simulink model "examen_simulacion_11_01_2024"  (R2024a)
settings: Solver=FixedStepAuto  StartTime=0.0  StopTime=10  FixedStep=0.01  RelTol=1e-3
values from neighbouring files (symbols this model uses):
  a_adelanto = y + Pd1_real    [examen_11_01_2024.m]
  a_adelanto2 = y2 + Pd1_real    [examen_11_01_2024.m]
  b_adelanto = abs(real(polos_LA(3)))    [examen_11_01_2024.m]
  b_adelanto2 = abs(real(polos_LA(2)))    [examen_11_01_2024.m]
  G_den = den    [examen_11_01_2024.m]
  G_num = num    [examen_11_01_2024.m]
  ganancias = 15:2:25    [examen_11_01_2024.m]
undefined symbols (not defined in the file or in its folder): K_rlocfind, K_rlocfind2
libraries: simulink x1
settings Model: Creator=david  LastModifiedBy=david

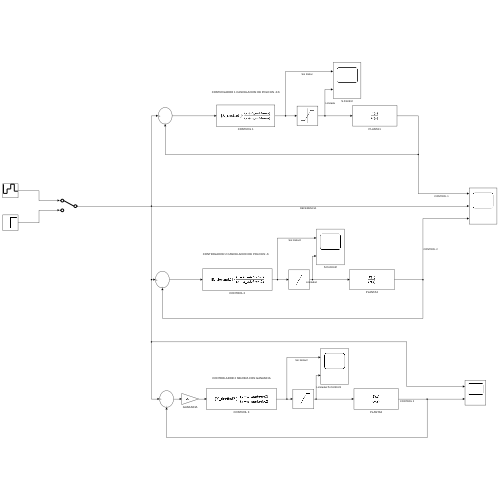
[thumbnail: Simulink's stored preview of the top-level diagram]
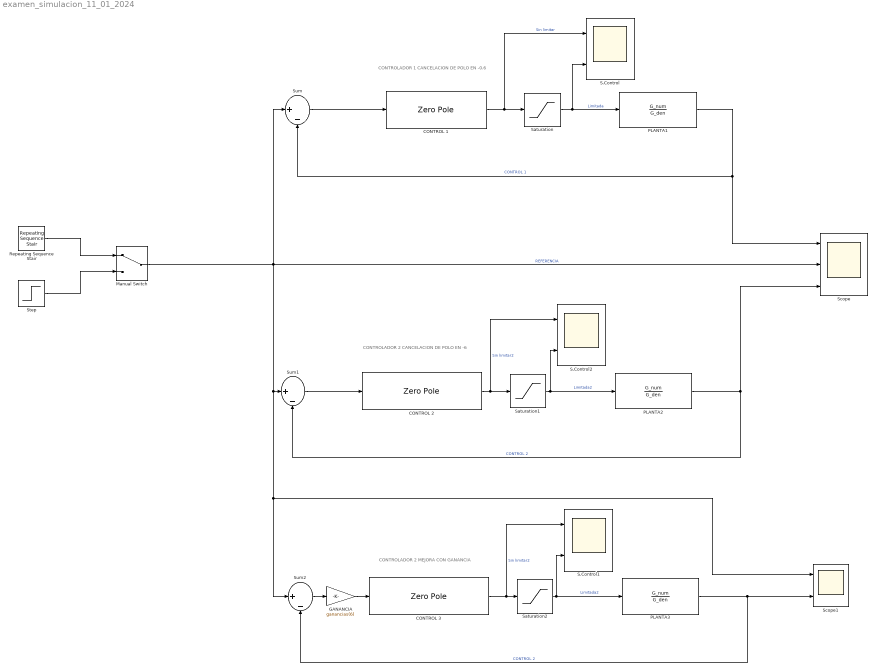
== system examen_simulacion_11_01_2024 ==
  note: CONTROLADOR 1 CANCELACION DE POLO EN -0.6
  note: CONTROLADOR 2 CANCELACION DE POLO EN -6
  note: CONTROLADOR 2 MEJORA CON GANANCIA
  CONTROL 1 : ZeroPole  Zeros=[-b_adelanto]  Poles=[-a_adelanto]  Gain=[K_rlocfind]
  CONTROL 2 : ZeroPole  Zeros=[-b_adelanto2]  Poles=[-a_adelanto2]  Gain=[K_rlocfind2]
  CONTROL 3 : ZeroPole  Zeros=[-b_adelanto2]  Poles=[-a_adelanto2]  Gain=[K_rlocfind2]
  GANANCIA : Gain  Gain=ganancias(6)
  Manual Switch : ManualSwitch
  PLANTA1 : TransferFcn  Numerator=G_num  Denominator=G_den
  PLANTA2 : TransferFcn  Numerator=G_num  Denominator=G_den
  PLANTA3 : TransferFcn  Numerator=G_num  Denominator=G_den
  Repeating Sequence Stair : simulink/Sources/Repeating Sequence Stair  OutValues=[1 3 5 2].'  tsamp=2  OutMin=[]  OutMax=[]  OutDataTypeStr=double  OutputDataTypeScalingMode=double  OutDataType=fixdt(0,8)  ConRadixGroup=Best Precision: Vector-wise  OutScaling=2^-12
  S.Control : Scope  NumInputPorts=2
  S.Control1 : Scope  NumInputPorts=2
  S.Control2 : Scope  NumInputPorts=2
  Saturation : Saturate  UpperLimit=10  LowerLimit=-10
  Saturation1 : Saturate  UpperLimit=10  LowerLimit=-10
  Saturation2 : Saturate  UpperLimit=10  LowerLimit=-10
  Scope : Scope  NumInputPorts=3
  Scope1 : Scope  NumInputPorts=2
  Step : Step  SampleTime=0
  Sum : Sum  Inputs=|+-
  Sum1 : Sum  Inputs=|+-
  Sum2 : Sum  Inputs=|+-
  wires:
  Sum/1 -> CONTROL 1/1
  PLANTA1/1 -> Scope/1, Sum/2  "CONTROL 1"
  Manual Switch/1 -> Sum1/1, Sum2/1, Scope1/1, Scope/2, Sum/1  "REFERENCIA"
  Repeating Sequence Stair/1 -> Manual Switch/1
  Step/1 -> Manual Switch/2
  CONTROL 1/1 -> S.Control/1, Saturation/1  "Sin limitar"
  Saturation/1 -> S.Control/2, PLANTA1/1  "Limitada"
  PLANTA2/1 -> Scope/3, Sum1/2  "CONTROL 2"
  CONTROL 2/1 -> S.Control2/1, Saturation1/1  "Sin limitar2"
  Saturation1/1 -> PLANTA2/1, S.Control2/2  "Limitada2"
  Sum1/1 -> CONTROL 2/1
  CONTROL 3/1 -> S.Control1/1, Saturation2/1  "Sin limitar2"
  Saturation2/1 -> PLANTA3/1, S.Control1/2  "Limitada2"
  PLANTA3/1 -> Sum2/2, Scope1/2  "CONTROL 2"
  Sum2/1 -> GANANCIA/1
  GANANCIA/1 -> CONTROL 3/1
